simulink model "Neurofeedback_PID_WithoutFNIRS"  (R2021a)
settings: Solver=VariableStepAuto  StartTime=0.0  StopTime=60  FixedStep=1/10.4  RelTol=1e-6
libraries: pid_lib x1
settings Model: EnablePacing=on  Creator=mdls3  LastModifiedBy=mdls3

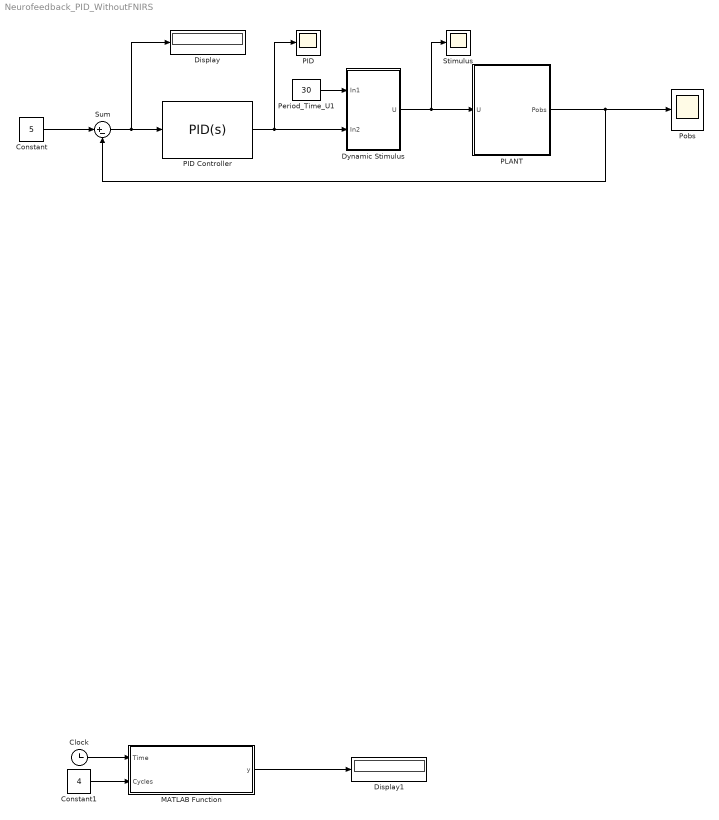
== system Neurofeedback_PID_WithoutFNIRS ==
  Clock : Clock
  Constant : Constant  Value=5
  Constant1 : Constant  Value=4
  Display : Display
  Display1 : Display
  Dynamic Stimulus : Subsystem
  MATLAB Function : MATLAB Function  TreatAsAtomicUnit=on
  PID : Scope
  PID Controller : pid_lib/PID Controller  Controller=PID  Form=Ideal  TimeDomain=Continuous-time  UseExternalTs=off  SampleTime=-1  IntegratorMethod=Forward Euler  FilterMethod=Forward Euler  ControllerParametersSource=internal  P=0.8725  I=0.1525  D=0.105  UseFilter=on  N=100  TunerSelectOption=Transfer Function Based (PID Tuner App)  InitialConditionSource=internal  InitialConditionForIntegrator=0  InitialConditionForFilter=0  DifferentiatorICPrevScaledInput=0  ExternalReset=none  TrackingMode=off  Kt=1  LimitOutput=off  SatLimitsSource=internal  UpperSaturationLimit=inf  LowerSaturationLimit=-inf  LinearizeAsGain=on  AntiWindupMode=none  Kb=1  POutMin=[]  POutMax=[]  IOutMin=[]  IOutMax=[]  DOutMin=[]  DOutMax=[]  NOutMin=[]  NOutMax=[]  SumOutMin=[]  SumOutMax=[]  SaturationOutMin=[]  SaturationOutMax=[]  PParamMin=[]  PParamMax=[]  IParamMin=[]  IParamMax=[]  DParamMin=[]  DParamMax=[]  NParamMin=[]  NParamMax=[]  KbParamMin=[]  KbParamMax=[]  KtParamMin=[]  KtParamMax=[]  KbOutMin=[]  KbOutMax=[]  KtOutMin=[]  KtOutMax=[]  IntegratorOutMin=[]  IntegratorOutMax=[]  FilterOutMin=[]  FilterOutMax=[]  SumI1OutMin=[]  SumI1OutMax=[]  SumI2OutMin=[]  SumI2OutMax=[]  SumI3OutMin=[]  SumI3OutMax=[]  SumI4OutMin=[]  SumI4OutMax=[]  SumDOutMin=[]  SumDOutMax=[]  DifferentiatorOutMin=[]  DifferentiatorOutMax=[]  FilterDiffOutCoefMin=[]  FilterDiffOutCoefMax=[]  ReciprocalOutMin=[]  ReciprocalOutMax=[]  SumDenOutMin=[]  SumDenOutMax=[]  SumNumOutMin=[]  SumNumOutMax=[]  DivideOutMin=[]  DivideOutMax=[]  UdiffTsProdOutMin=[]  UdiffTsProdOutMax=[]  NTsProdOutMin=[]  NTsProdOutMax=[]  UintegralTsProdOutMin=[]  UintegralTsProdOutMax=[]  UngainTsProdOutMin=[]  UngainTsProdOutMax=[]  IntegratorContinuousStateAttributes=''  IntegratorStateMustResolveToSignalObject=off  IntegratorRTWStateStorageClass=Auto  FilterContinuousStateAttributes=''  FilterStateMustResolveToSignalObject=off  FilterRTWStateStorageClass=Auto  ParallelPVariant=Passthrough  IdealPVariant=InternalParameters  IVariant=InternalParameters  DVariant=InternalParameters  IntegratorVariant=Continuous  SatVariant=Disabled  AWVariant=Passthrough  PCopyVariant=Disabled  TRVariant=Disabled  FdbkBlocksVariant=Forward  IdealPFdbkVariant=Disabled  SatFdbkVariant=Disabled  DerivativeFilterVariant=ContFilter  NVariant=InternalParameters  NCopyVariant=Disabled  FilterICVariant=InternalICsFilter  IntegratorICVariant=InternalICs  ExternalResetVariant=Disabled  TRSumVariant=Passthrough  SumFdbkVariant=Disabled  SumVariant=Sum_PID  TsampFilterVariant=InternalTs  TsampNgainVariant=Passthrough  TsampIntegralVariant=Passthrough  ExternalSaturationOutDataTypeStr=Inherit: Same as second input
  PLANT : Subsystem
  Period_Time_U1 : Constant  Value=30
  Pobs : Scope
  Stimulus : Scope
  Sum : Sum  Inputs=|+-
  wires:
  Period_Time_U1/1 -> Dynamic Stimulus/1(In1)
  Dynamic Stimulus/1(U) -> Stimulus/1, PLANT/1(U)
  PID Controller/1 -> Dynamic Stimulus/2(In2), PID/1
  Sum/1 -> PID Controller/1, Display/1
  PLANT/1(Pobs) -> Pobs/1, Sum/2
  MATLAB Function/1(y) -> Display1/1
  Clock/1 -> MATLAB Function/1(Time)
  Constant1/1 -> MATLAB Function/2(Cycles)
  Constant/1 -> Sum/1

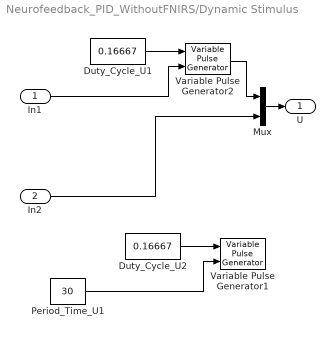
== system Neurofeedback_PID_WithoutFNIRS/Dynamic Stimulus ==
  In1 : Inport
  In2 : Inport  Port=2
  Duty_Cycle_U1 : Constant  Value=0.16667  OutMin=[0]  OutMax=[0.8]
  Duty_Cycle_U2 : Constant  Value=0.16667  OutMin=[0]  OutMax=[0.8]
  Mux : Mux  Inputs=2
  Period_Time_U1 : Constant  Value=30
  Variable Pulse Generator1 : VariablePulseGenerator  RunAtFixedTimeIntervals=on  SampleTime=1/10.4
  Variable Pulse Generator2 : VariablePulseGenerator  RunAtFixedTimeIntervals=on  SampleTime=1/10.4
  U : Outport
  wires:
  In1/1 -> Variable Pulse Generator2/2
  Mux/1 -> U/1
  Variable Pulse Generator2/1 -> Mux/1
  Duty_Cycle_U1/1 -> Variable Pulse Generator2/1
  Period_Time_U1/1 -> Variable Pulse Generator1/2
  Duty_Cycle_U2/1 -> Variable Pulse Generator1/1
  In2/1 -> Mux/2

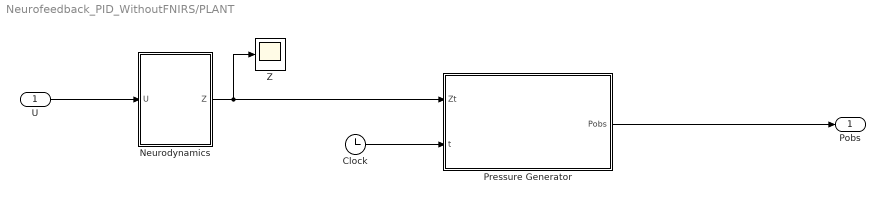
== system Neurofeedback_PID_WithoutFNIRS/PLANT ==
  U : Inport
  Clock : Clock
  Neurodynamics : Subsystem
  Pressure Generator : MATLAB Function  TreatAsAtomicUnit=on
  Z : Scope
  Pobs : Outport
  wires:
  U/1 -> Neurodynamics/1(U)
  Clock/1 -> Pressure Generator/2(t)
  Pressure Generator/1(Pobs) -> Pobs/1
  Neurodynamics/1(Z) -> Pressure Generator/1(Zt), Z/1

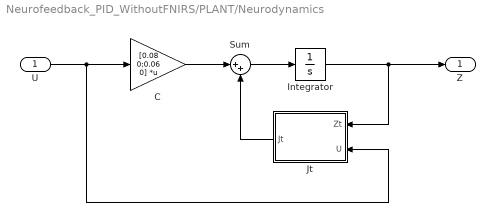
== system Neurofeedback_PID_WithoutFNIRS/PLANT/Neurodynamics ==
  U : Inport
  C : Gain  Gain=[0.08 0;0.06 0]  Multiplication=Matrix(K*u) (u vector)
  Integrator : Integrator
  Jt : MATLAB Function  TreatAsAtomicUnit=on
  Sum : Sum  Inputs=|++
  Z : Outport
  wires:
  Integrator/1 -> Jt/1(Zt), Z/1
  C/1 -> Sum/1
  Jt/1(Jt) -> Sum/2
  U/1 -> C/1, Jt/2(U)
  Sum/1 -> Integrator/1

== matlab function Neurofeedback_PID_WithoutFNIRS/PLANT/Neurodynamics/Jt ==
  data: Zt input; U input; Jt output
function Jt = fcn(Zt, U)
   A = [-0.16 -0.49;-0.02 -0.33];
   nRegions  = size(A,1);
   M = size(U,1); %nStimuli
   simulationLength = size(U,2);
   B = zeros(2,2,2);
   B1 = [0 0; 0 0]; %There must be a B per stimulus
   B2 = [-0.02 -0.77; 0.33 -1.31];
   B(:,:,1) = B1;
   B(:,:,2) = B2;
      assert(M == size(B,3),...
       'Unexpected number of induced connectivity parameters B.');
   T = zeros(nRegions); %nRegions x nRegions
    for t = 1:simulationLength
           for uu = 1:M % Sum (Uj * Bj)
               tmp = U(uu,t)*B(:,:,uu);
               T = -0.5*exp(T + tmp);  
           end
    end
Jt = (A*Zt) + (T*Zt);

== matlab function Neurofeedback_PID_WithoutFNIRS/MATLAB Function ==
  settings: updateMethod=DISCRETE
  data: y output; Time input; Cycles input
function y = Random_Setpoint(Time,Cycles)



min = 1; max = 6;
z = min + ((max-min).*(rand));
y = z;

== matlab function Neurofeedback_PID_WithoutFNIRS/PLANT/Pressure Generator ==
  data: Zt input; Pobs output; t input
function Pobs = fcn(Zt, t)
    R=28.2; %Resistor [Ohms];
    C=0.8; %Capacitor [Faradays];
    V= Zt(1,:); %Voltage or system reference;
    Vc = V * (exp(-t/(R*C))); % Voltage at the capacitor  
    
Pobs = Vc;
